simulink library "DoubletsLib"  (R2024b)
settings: Solver=VariableStepAuto  StartTime=0.0  StopTime=10.0  RelTol=1e-3
undefined symbols (not defined in the file): SimPar
libraries: simulink x15
settings Model: Creator=tbritton  LastModifiedBy=macheson
settings SolverCC: AlgebraicLoopSolver=TrustRegion
settings OptimizationCC: ReuseModelBlockBuffer=off
settings DebuggingCC: UnconnectedInputMsg=warning  UnconnectedOutputMsg=warning  UnconnectedLineMsg=warning
settings ModelReferenceCC: EnableRefExpFcnMdlSchedulingChecks=on
settings RTWCC: GPUComputeCapability=3.5  DLArmComputeVersion=19.05

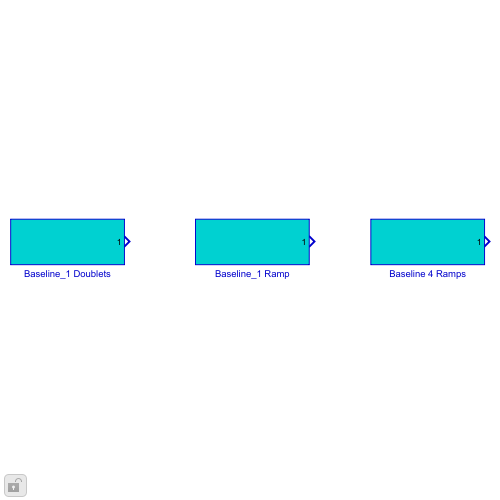
[thumbnail: Simulink's stored preview of the top-level diagram]
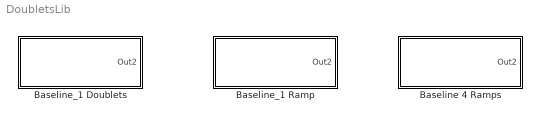
== system DoubletsLib ==
  Baseline 4 Ramps : Subsystem
  Baseline_1 Doublets : Subsystem
  Baseline_1 Ramp : Subsystem

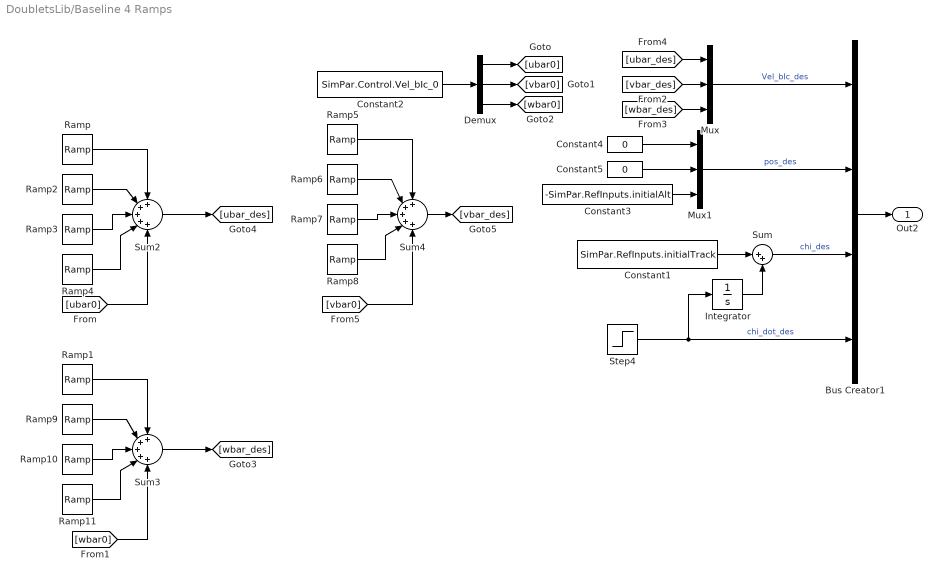
== system DoubletsLib/Baseline 4 Ramps ==
  Bus Creator1 : BusCreator  Inputs=4  OutDataTypeStr=Bus: BUS_REF_INPUT
  Constant1 : Constant  Value=SimPar.RefInputs.initialTrack
  Constant2 : Constant  Value=SimPar.Control.Vel_bIc_0
  Constant3 : Constant  Value=-SimPar.RefInputs.initialAlt
  Constant4 : Constant  Value=0
  Constant5 : Constant  Value=0
  Demux : Demux  Outputs=3
  Integrator : Integrator
  Mux : Mux  Inputs=3
  Mux1 : Mux  Inputs=3
  Ramp : simulink/Sources/Ramp  slope=SimPar.RefInputs.ramps.Vel_slope1(1)  start=SimPar.RefInputs.ramps.Vel_startTime1(1)  InitialOutput=SimPar.RefInputs.ramps.Vel_initialValue1(1)
  Ramp1 : simulink/Sources/Ramp  slope=SimPar.RefInputs.ramps.Vel_slope1(3)  start=SimPar.RefInputs.ramps.Vel_startTime1(3)  InitialOutput=SimPar.RefInputs.ramps.Vel_initialValue1(3)
  Ramp10 : simulink/Sources/Ramp  slope=SimPar.RefInputs.ramps.Vel_slope3(3)  start=SimPar.RefInputs.ramps.Vel_startTime3(3)  InitialOutput=SimPar.RefInputs.ramps.Vel_initialValue3(3)
  Ramp11 : simulink/Sources/Ramp  slope=SimPar.RefInputs.ramps.Vel_slope4(3)  start=SimPar.RefInputs.ramps.Vel_startTime4(3)  InitialOutput=SimPar.RefInputs.ramps.Vel_initialValue4(3)
  Ramp2 : simulink/Sources/Ramp  slope=SimPar.RefInputs.ramps.Vel_slope2(1)  start=SimPar.RefInputs.ramps.Vel_startTime2(1)  InitialOutput=SimPar.RefInputs.ramps.Vel_initialValue2(1)
  Ramp3 : simulink/Sources/Ramp  slope=SimPar.RefInputs.ramps.Vel_slope3(1)  start=SimPar.RefInputs.ramps.Vel_startTime3(1)  InitialOutput=SimPar.RefInputs.ramps.Vel_initialValue3(1)
  Ramp4 : simulink/Sources/Ramp  slope=SimPar.RefInputs.ramps.Vel_slope4(1)  start=SimPar.RefInputs.ramps.Vel_startTime4(1)  InitialOutput=SimPar.RefInputs.ramps.Vel_initialValue4(1)
  Ramp5 : simulink/Sources/Ramp  slope=SimPar.RefInputs.ramps.Vel_slope1(2)  start=SimPar.RefInputs.ramps.Vel_startTime1(2)  InitialOutput=SimPar.RefInputs.ramps.Vel_initialValue1(2)
  Ramp6 : simulink/Sources/Ramp  slope=SimPar.RefInputs.ramps.Vel_slope2(2)  start=SimPar.RefInputs.ramps.Vel_startTime2(2)  InitialOutput=SimPar.RefInputs.ramps.Vel_initialValue2(2)
  Ramp7 : simulink/Sources/Ramp  slope=SimPar.RefInputs.ramps.Vel_slope3(2)  start=SimPar.RefInputs.ramps.Vel_startTime3(2)  InitialOutput=SimPar.RefInputs.ramps.Vel_initialValue3(2)
  Ramp8 : simulink/Sources/Ramp  slope=SimPar.RefInputs.ramps.Vel_slope4(2)  start=SimPar.RefInputs.ramps.Vel_startTime4(2)  InitialOutput=SimPar.RefInputs.ramps.Vel_initialValue4(2)
  Ramp9 : simulink/Sources/Ramp  slope=SimPar.RefInputs.ramps.Vel_slope2(3)  start=SimPar.RefInputs.ramps.Vel_startTime2(3)  InitialOutput=SimPar.RefInputs.ramps.Vel_initialValue2(3)
  Step4 : Step  Time=SimPar.RefInputs.doublets.Track_stepTime  Before=SimPar.RefInputs.doublets.Track_initialValue  After=SimPar.RefInputs.doublets.Track_finalValue  SampleTime=0
  Sum : Sum  Inputs=|++
  Sum2 : Sum  Inputs=+++++
  Sum3 : Sum  Inputs=+++++
  Sum4 : Sum  Inputs=+++++
  Out2 : Outport
  wires:
  Constant5/1 -> Mux1/2
  Constant4/1 -> Mux1/1
  Constant3/1 -> Mux1/3
  Ramp/1 -> Sum2/1
  Integrator/1 -> Sum/2
  Sum/1 -> Bus Creator1/3  "chi_des"
  Sum2/1 -> [ubar_des]
  [ubar_des] -> Mux/1
  [wbar_des] -> Mux/3
  Constant1/1 -> Sum/1
  Step4/1 -> Bus Creator1/4, Integrator/1  "chi_dot_des"
  [vbar_des] -> Mux/2
  [ubar0] -> Sum2/5
  Bus Creator1/1 -> Out2/1
  Mux/1 -> Bus Creator1/1  "Vel_bIc_des"
  Mux1/1 -> Bus Creator1/2  "pos_des"
  Demux/1 -> [ubar0]
  Demux/3 -> [wbar0]
  Demux/2 -> [vbar0]
  Constant2/1 -> Demux/1
  Ramp2/1 -> Sum2/2
  Ramp3/1 -> Sum2/3
  Ramp4/1 -> Sum2/4
  [vbar0] -> Sum4/5
  Sum4/1 -> [vbar_des]
  [wbar0] -> Sum3/5
  Sum3/1 -> [wbar_des]
  Ramp5/1 -> Sum4/1
  Ramp6/1 -> Sum4/2
  Ramp7/1 -> Sum4/3
  Ramp8/1 -> Sum4/4
  Ramp11/1 -> Sum3/4
  Ramp10/1 -> Sum3/3
  Ramp9/1 -> Sum3/2
  Ramp1/1 -> Sum3/1

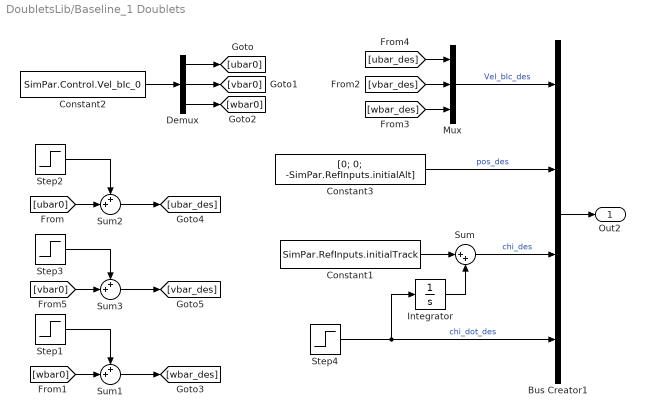
== system DoubletsLib/Baseline_1 Doublets ==
  Bus Creator1 : BusCreator  Inputs=4  OutDataTypeStr=Bus: BUS_REF_INPUT
  Constant1 : Constant  Value=SimPar.RefInputs.initialTrack
  Constant2 : Constant  Value=SimPar.Control.Vel_bIc_0
  Constant3 : Constant  Value=[0; 0; -SimPar.RefInputs.initialAlt]
  Demux : Demux  Outputs=3
  Integrator : Integrator
  Mux : Mux  Inputs=3
  Step1 : Step  Time=SimPar.RefInputs.doublets.Vel_stepTime(3)  Before=SimPar.RefInputs.doublets.Vel_initialValue(3)  After=SimPar.RefInputs.doublets.Vel_finalValue(3)  SampleTime=0
  Step2 : Step  Time=SimPar.RefInputs.doublets.Vel_stepTime(1)  Before=SimPar.RefInputs.doublets.Vel_initialValue(1)  After=SimPar.RefInputs.doublets.Vel_finalValue(1)  SampleTime=0
  Step3 : Step  Time=SimPar.RefInputs.doublets.Vel_stepTime(2)  Before=SimPar.RefInputs.doublets.Vel_initialValue(2)  After=SimPar.RefInputs.doublets.Vel_finalValue(2)  SampleTime=0
  Step4 : Step  Time=SimPar.RefInputs.doublets.Track_stepTime  Before=SimPar.RefInputs.doublets.Track_initialValue  After=SimPar.RefInputs.doublets.Track_finalValue  SampleTime=0
  Sum : Sum  Inputs=|++
  Sum1 : Sum  Inputs=++|
  Sum2 : Sum  Inputs=++|
  Sum3 : Sum  Inputs=++|
  Out2 : Outport
  wires:
  Constant2/1 -> Demux/1
  Demux/2 -> [vbar0]
  Demux/3 -> [wbar0]
  Sum1/1 -> [wbar_des]
  Demux/1 -> [ubar0]
  Constant3/1 -> Bus Creator1/2  "pos_des"
  Mux/1 -> Bus Creator1/1  "Vel_bIc_des"
  Bus Creator1/1 -> Out2/1
  [ubar0] -> Sum2/2
  [wbar0] -> Sum1/2
  [vbar_des] -> Mux/2
  Step4/1 -> Integrator/1, Bus Creator1/4  "chi_dot_des"
  Constant1/1 -> Sum/1
  [wbar_des] -> Mux/3
  [ubar_des] -> Mux/1
  Sum2/1 -> [ubar_des]
  [vbar0] -> Sum3/2
  Sum3/1 -> [vbar_des]
  Sum/1 -> Bus Creator1/3  "chi_des"
  Integrator/1 -> Sum/2
  Step1/1 -> Sum1/1
  Step3/1 -> Sum3/1
  Step2/1 -> Sum2/1

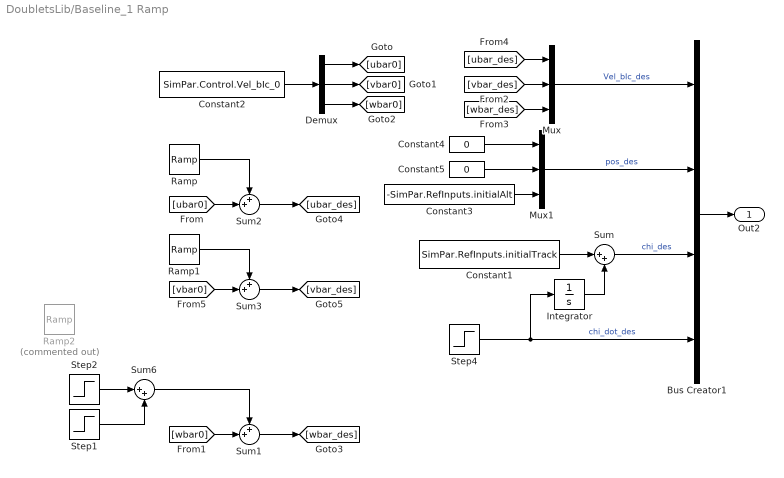
== system DoubletsLib/Baseline_1 Ramp ==
  Bus Creator1 : BusCreator  Inputs=4  OutDataTypeStr=Bus: BUS_REF_INPUT
  Constant1 : Constant  Value=SimPar.RefInputs.initialTrack
  Constant2 : Constant  Value=SimPar.Control.Vel_bIc_0
  Constant3 : Constant  Value=-SimPar.RefInputs.initialAlt
  Constant4 : Constant  Value=0
  Constant5 : Constant  Value=0
  Demux : Demux  Outputs=3
  Integrator : Integrator
  Mux : Mux  Inputs=3
  Mux1 : Mux  Inputs=3
  Ramp : simulink/Sources/Ramp  slope=SimPar.RefInputs.ramps.Vel_slope(1)  start=SimPar.RefInputs.ramps.Vel_startTime(1)  InitialOutput=SimPar.RefInputs.ramps.Vel_initialValue(1)
  Ramp1 : simulink/Sources/Ramp  slope=SimPar.RefInputs.ramps.Vel_slope(2)  start=SimPar.RefInputs.ramps.Vel_startTime(2)  InitialOutput=SimPar.RefInputs.ramps.Vel_initialValue(2)
  Ramp2 : simulink/Sources/Ramp  Commented=on  slope=SimPar.RefInputs.ramps.Vel_slope(3)  start=SimPar.RefInputs.ramps.Vel_startTime(3)  InitialOutput=SimPar.RefInputs.ramps.Vel_initialValue(3)
  Step1 : Step  Time=SimPar.RefInputs.doublets.Vel_stepTime(3)+50  Before=SimPar.RefInputs.doublets.Vel_initialValue(3)  After=-SimPar.RefInputs.doublets.Vel_finalValue(3)  SampleTime=0
  Step2 : Step  Time=SimPar.RefInputs.doublets.Vel_stepTime(3)  Before=SimPar.RefInputs.doublets.Vel_initialValue(3)  After=SimPar.RefInputs.doublets.Vel_finalValue(3)  SampleTime=0
  Step4 : Step  Time=SimPar.RefInputs.doublets.Track_stepTime  Before=SimPar.RefInputs.doublets.Track_initialValue  After=SimPar.RefInputs.doublets.Track_finalValue  SampleTime=0
  Sum : Sum  Inputs=|++
  Sum1 : Sum  Inputs=++|
  Sum2 : Sum  Inputs=++|
  Sum3 : Sum  Inputs=++|
  Sum6 : Sum  Inputs=|++
  Out2 : Outport
  wires:
  Constant2/1 -> Demux/1
  Demux/2 -> [vbar0]
  Demux/3 -> [wbar0]
  Sum1/1 -> [wbar_des]
  Demux/1 -> [ubar0]
  Mux1/1 -> Bus Creator1/2  "pos_des"
  Mux/1 -> Bus Creator1/1  "Vel_bIc_des"
  Bus Creator1/1 -> Out2/1
  [ubar0] -> Sum2/2
  [wbar0] -> Sum1/2
  [vbar_des] -> Mux/2
  Step4/1 -> Integrator/1, Bus Creator1/4  "chi_dot_des"
  Constant1/1 -> Sum/1
  [wbar_des] -> Mux/3
  [ubar_des] -> Mux/1
  Sum2/1 -> [ubar_des]
  [vbar0] -> Sum3/2
  Sum3/1 -> [vbar_des]
  Sum/1 -> Bus Creator1/3  "chi_des"
  Integrator/1 -> Sum/2
  Sum6/1 -> Sum1/1
  Ramp1/1 -> Sum3/1
  Ramp/1 -> Sum2/1
  Step2/1 -> Sum6/1
  Step1/1 -> Sum6/2
  Constant3/1 -> Mux1/3
  Constant4/1 -> Mux1/1
  Constant5/1 -> Mux1/2
